simulink model "finalProjectLuenberger"  (R2015b)
settings: Solver=VariableStepAuto  StartTime=0.0  StopTime=20  RelTol=1e-3
undefined symbols (not defined in the file): C, L, l1, l2, M, m1, m2, X0, X_est, Xhat0
settings Model: Creator=Rishabh  LastModifiedBy=Rishabh
settings DataIOCC: LimitDataPoints=off
settings DebuggingCC: AllowSymbolicDim=on
settings ModelReferenceCC: PropagateSignalLabelsOutOfModel=on
settings GRTTargetCC: GeneratePreprocessorConditionals=Disable all

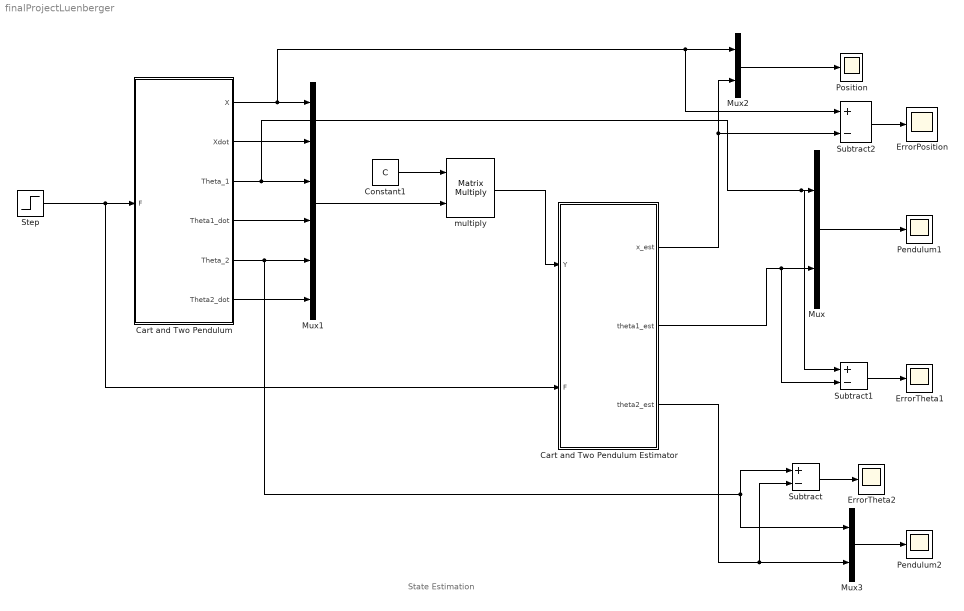
== system finalProjectLuenberger ==
  note: State Estimation
  "Cart and Two Pendulum " : Subsystem
  Cart and Two Pendulum Estimator : Subsystem
  Constant1 : Constant  Value=C  VectorParams1D=off
  ErrorPosition : Scope
  ErrorTheta1 : Scope
  ErrorTheta2 : Scope
  Mux : Mux  Inputs=2
  Mux1 : Mux  Inputs=6
  Mux2 : Mux  Inputs=2
  Mux3 : Mux  Inputs=2
  Pendulum1 : Scope
  Pendulum2 : Scope
  Position : Scope
  Step : Step  After=1000  SampleTime=0
  Subtract : Sum  Inputs=+-
  Subtract1 : Sum  Inputs=+-
  Subtract2 : Sum  Inputs=+-
  multiply : Product  Inputs=**  Multiplication=Matrix(*)
  wires:
  Mux/1 -> Pendulum1/1
  "Cart and Two Pendulum "/1(X) -> Mux2/1, Subtract2/1, Mux1/1
  "Cart and Two Pendulum "/2(Xdot) -> Mux1/2
  "Cart and Two Pendulum "/3(Theta_1) -> Mux1/3, Subtract1/1, Mux/1
  "Cart and Two Pendulum "/4(Theta1_dot) -> Mux1/4
  "Cart and Two Pendulum "/5(Theta_2) -> Mux3/1, Subtract/1, Mux1/5
  "Cart and Two Pendulum "/6(Theta2_dot) -> Mux1/6
  multiply/1 -> Cart and Two Pendulum Estimator/1(Y)
  Step/1 -> Cart and Two Pendulum Estimator/2(F), "Cart and Two Pendulum "/1(F)
  Cart and Two Pendulum Estimator/1(x_est) -> Subtract2/2, Mux2/2
  Mux2/1 -> Position/1
  Cart and Two Pendulum Estimator/2(theta1_est) -> Subtract1/2, Mux/2
  Cart and Two Pendulum Estimator/3(theta2_est) -> Mux3/2, Subtract/2
  Mux3/1 -> Pendulum2/1
  Constant1/1 -> multiply/1
  Mux1/1 -> multiply/2
  Subtract/1 -> ErrorTheta2/1
  Subtract1/1 -> ErrorTheta1/1
  Subtract2/1 -> ErrorPosition/1

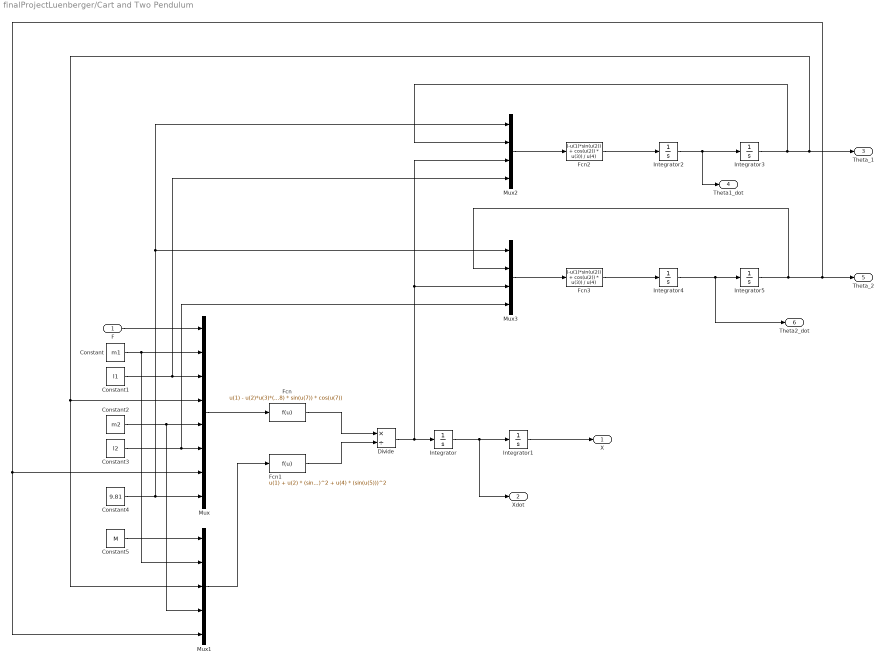
== system finalProjectLuenberger/Cart and Two Pendulum  ==
  F : Inport
  Constant : Constant  Value=m1
  Constant1 : Constant  Value=l1
  Constant2 : Constant  Value=m2
  Constant3 : Constant  Value=l2
  Constant4 : Constant  Value=9.81
  Constant5 : Constant  Value=M
  Divide : Product  Inputs=*/
  Fcn : Fcn  Expr=u(1) - u(2)*u(3)*(u(4)^2)*sin(u(4)) - u(5) * u(6) * (u(7)^2)*sin(u(7))-u(2)*u(8)*sin(u(4))*cos(u(4)) - u(5) * u(8) * sin(u(7)) * cos(u(7))
  Fcn1 : Fcn  Expr=u(1) + u(2) * (sin(u(3)))^2 + u(4) * (sin(u(5)))^2
  Fcn2 : Fcn  Expr=(-u(1)*sin(u(2)) + cos(u(2)) * u(3)) / u(4)
  Fcn3 : Fcn  Expr=(-u(1)*sin(u(2)) + cos(u(2)) * u(3)) / u(4)
  Integrator : Integrator
  Integrator1 : Integrator  InitialCondition=X0(1)
  Integrator2 : Integrator
  Integrator3 : Integrator  InitialCondition=X0(3)
  Integrator4 : Integrator
  Integrator5 : Integrator  InitialCondition=X0(5)
  Mux : Mux  Inputs=8
  Mux1 : Mux  Inputs=5
  Mux2 : Mux
  Mux3 : Mux
  X : Outport
  Xdot : Outport  Port=2
  Theta_1 : Outport  Port=3
  Theta1_dot : Outport  Port=4
  Theta_2 : Outport  Port=5
  Theta2_dot : Outport  Port=6
  wires:
  Mux1/1 -> Fcn1/1
  Mux3/1 -> Fcn3/1
  Fcn/1 -> Divide/1
  Integrator2/1 -> Theta1_dot/1, Integrator3/1
  Integrator4/1 -> Theta2_dot/1, Integrator5/1
  Integrator5/1 -> Theta_2/1, Mux/7, Mux1/5, Mux3/2
  Integrator3/1 -> Mux2/2, Theta_1/1, Mux1/3, Mux/4
  Divide/1 -> Mux3/3, Mux2/3, Integrator/1
  Constant5/1 -> Mux1/1
  Constant3/1 -> Mux3/4, Mux/6
  Constant2/1 -> Mux1/4, Mux/5
  Constant/1 -> Mux1/2, Mux/2
  F/1 -> Mux/1
  Constant1/1 -> Mux2/4, Mux/3
  Integrator/1 -> Xdot/1, Integrator1/1
  Fcn2/1 -> Integrator2/1
  Constant4/1 -> Mux2/1, Mux3/1, Mux/8
  Mux2/1 -> Fcn2/1
  Integrator1/1 -> X/1
  Mux/1 -> Fcn/1
  Fcn3/1 -> Integrator4/1
  Fcn1/1 -> Divide/2

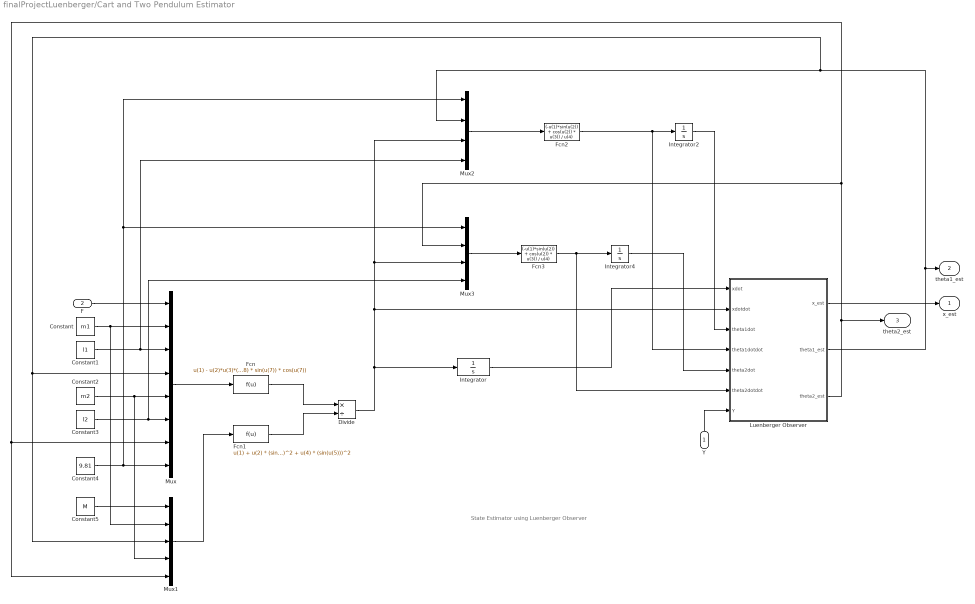
== system finalProjectLuenberger/Cart and Two Pendulum Estimator ==
  note: State Estimator using Luenberger Observer
  Y : Inport
  F : Inport  Port=2
  Constant : Constant  Value=m1
  Constant1 : Constant  Value=l1
  Constant2 : Constant  Value=m2
  Constant3 : Constant  Value=l2
  Constant4 : Constant  Value=9.81
  Constant5 : Constant  Value=M
  Divide : Product  Inputs=*/
  Fcn : Fcn  Expr=u(1) - u(2)*u(3)*(u(4)^2)*sin(u(4)) - u(5) * u(6) * (u(7)^2)*sin(u(7))-u(2)*u(8)*sin(u(4))*cos(u(4)) - u(5) * u(8) * sin(u(7)) * cos(u(7))
  Fcn1 : Fcn  Expr=u(1) + u(2) * (sin(u(3)))^2 + u(4) * (sin(u(5)))^2
  Fcn2 : Fcn  Expr=(-u(1)*sin(u(2)) + cos(u(2)) * u(3)) / u(4)
  Fcn3 : Fcn  Expr=(-u(1)*sin(u(2)) + cos(u(2)) * u(3)) / u(4)
  Integrator : Integrator  InitialCondition=X_est(1)
  Integrator2 : Integrator  InitialCondition=X_est(3)
  Integrator4 : Integrator  InitialCondition=X_est(5)
  Luenberger Observer : Subsystem
  Mux : Mux  Inputs=8
  Mux1 : Mux  Inputs=5
  Mux2 : Mux
  Mux3 : Mux
  x_est : Outport
  theta1_est : Outport  Port=2
  theta2_est : Outport  Port=3
  wires:
  Fcn1/1 -> Divide/2
  Fcn3/1 -> Luenberger Observer/6(theta2dotdot), Integrator4/1
  Mux/1 -> Fcn/1
  Mux2/1 -> Fcn2/1
  Constant4/1 -> Mux/8, Mux3/1, Mux2/1
  Fcn2/1 -> Luenberger Observer/4(theta1dotdot), Integrator2/1
  Constant1/1 -> Mux/3, Mux2/4
  F/1 -> Mux/1
  Constant/1 -> Mux/2, Mux1/2
  Constant2/1 -> Mux/5, Mux1/4
  Constant3/1 -> Mux/6, Mux3/4
  Constant5/1 -> Mux1/1
  Divide/1 -> Luenberger Observer/2(xdotdot), Mux2/3, Mux3/3, Integrator/1
  Fcn/1 -> Divide/1
  Mux3/1 -> Fcn3/1
  Mux1/1 -> Fcn1/1
  Luenberger Observer/3(theta2_est) -> theta2_est/1, Mux1/5, Mux/7, Mux3/2
  Luenberger Observer/2(theta1_est) -> theta1_est/1, Mux1/3, Mux/4, Mux2/2
  Y/1 -> Luenberger Observer/7(Y)
  Luenberger Observer/1(x_est) -> x_est/1
  Integrator/1 -> Luenberger Observer/1("xdot ")
  Integrator2/1 -> Luenberger Observer/3(theta1dot)
  Integrator4/1 -> Luenberger Observer/5(theta2dot)

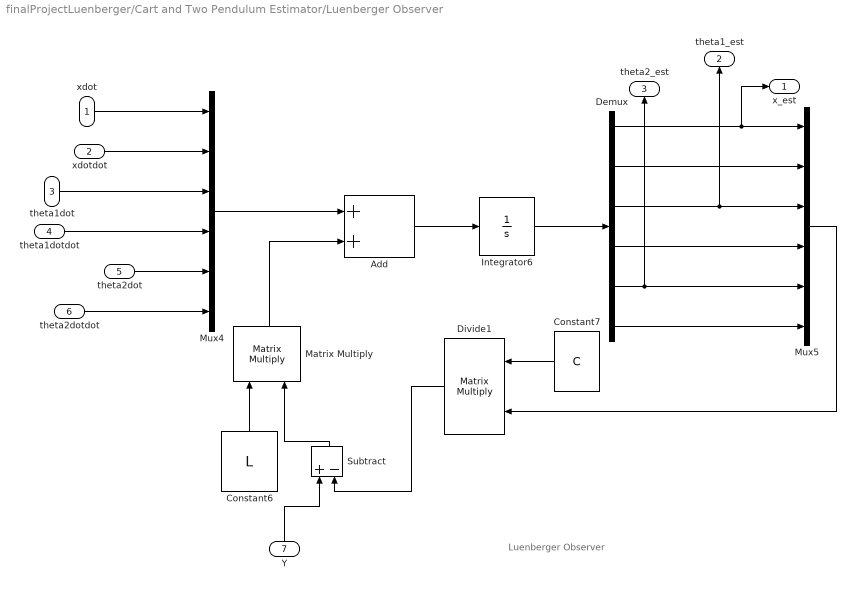
== system finalProjectLuenberger/Cart and Two Pendulum Estimator/Luenberger Observer ==
  note: Luenberger Observer
  "xdot " : Inport
  xdotdot : Inport  Port=2
  theta1dot : Inport  Port=3
  theta1dotdot : Inport  Port=4
  theta2dot : Inport  Port=5
  theta2dotdot : Inport  Port=6
  Y : Inport  Port=7
  Add : Sum
  Constant6 : Constant  Value=L
  Constant7 : Constant  Value=C  VectorParams1D=off
  Demux : Demux  Outputs=6
  Divide1 : Product  Inputs=**  Multiplication=Matrix(*)
  Integrator6 : Integrator  InitialCondition=Xhat0
  Matrix Multiply : Product  Multiplication=Matrix(*)
  Mux4 : Mux  Inputs=6
  Mux5 : Mux  Inputs=6
  Subtract : Sum  Inputs=+-
  x_est : Outport
  theta1_est : Outport  Port=2
  theta2_est : Outport  Port=3
  wires:
  Demux/4 -> Mux5/4
  Mux4/1 -> Add/1
  Demux/1 -> Mux5/1, x_est/1
  Demux/2 -> Mux5/2
  Demux/6 -> Mux5/6
  Integrator6/1 -> Demux/1
  Add/1 -> Integrator6/1
  Demux/3 -> Mux5/3, theta1_est/1
  Divide1/1 -> Subtract/2
  Matrix Multiply/1 -> Add/2
  Subtract/1 -> Matrix Multiply/2
  Y/1 -> Subtract/1
  Constant7/1 -> Divide1/1
  Demux/5 -> Mux5/5, theta2_est/1
  Mux5/1 -> Divide1/2
  Constant6/1 -> Matrix Multiply/1
  "xdot "/1 -> Mux4/1
  xdotdot/1 -> Mux4/2
  theta1dot/1 -> Mux4/3
  theta1dotdot/1 -> Mux4/4
  theta2dot/1 -> Mux4/5
  theta2dotdot/1 -> Mux4/6
